simulink model "O4"  (R2020b)
settings: Solver=ode4  StartTime=0.0  StopTime=180  FixedStep=0.005  MinStep=0.001  RelTol=1e-3
model workspace (MAT data in the model file):
  Optimisation01_sdosession = sldodialogs.data.SessionData
  Optimisation01_sdosession.Version = '3.0'
  Optimisation01_sdosession.Data.ModelName = 'Optimisation01'
  Optimisation01_sdosession.Data.ToolType = 'ResponseOptimization'
  Optimisation01_sdosession.Data.GUIOptions.NoPromptClose = 0
  Optimisation01_sdosession.Data.Workspace.LocalWorkspace.DesignVars(1) = param.Continuous
  Optimisation01_sdosession.Data.Workspace.LocalWorkspace.DesignVars(1).Scale_ = 128
  Optimisation01_sdosession.Data.Workspace.LocalWorkspace.DesignVars(1).Size_ = [1 1]
  Optimisation01_sdosession.Data.Workspace.LocalWorkspace.DesignVars(1).Value_ = 50.1084192258
  Optimisation01_sdosession.Data.Workspace.LocalWorkspace.DesignVars(1).pID = paramid.Variable
  Optimisation01_sdosession.Data.Workspace.LocalWorkspace.DesignVars(1).pID.Name = 'Kd'
  Optimisation01_sdosession.Data.Workspace.LocalWorkspace.DesignVars(2) = param.Continuous
  Optimisation01_sdosession.Data.Workspace.LocalWorkspace.DesignVars(2).Scale_ = 8
  Optimisation01_sdosession.Data.Workspace.LocalWorkspace.DesignVars(2).Size_ = [1 1]
  Optimisation01_sdosession.Data.Workspace.LocalWorkspace.DesignVars(2).Value_ = 6.29568850936
  Optimisation01_sdosession.Data.Workspace.LocalWorkspace.DesignVars(2).pID = paramid.Variable
  Optimisation01_sdosession.Data.Workspace.LocalWorkspace.DesignVars(2).pID.Name = 'Ki'
  Optimisation01_sdosession.Data.Workspace.LocalWorkspace.DesignVars(3) = param.Continuous
  Optimisation01_sdosession.Data.Workspace.LocalWorkspace.DesignVars(3).Scale_ = 512
  Optimisation01_sdosession.Data.Workspace.LocalWorkspace.DesignVars(3).Size_ = [1 1]
  Optimisation01_sdosession.Data.Workspace.LocalWorkspace.DesignVars(3).Value_ = 364.260452278
  Optimisation01_sdosession.Data.Workspace.LocalWorkspace.DesignVars(3).pID = paramid.Variable
  Optimisation01_sdosession.Data.Workspace.LocalWorkspace.DesignVars(3).pID.Name = 'Kp'
  Optimisation01_sdosession.Data.Workspace.LocalWorkspace.ReqValues.Name = 'SignalProperty'
  Optimisation01_sdosession.Data.Workspace.LocalWorkspace.ReqValues.Type = 'min'
  Optimisation01_sdosession.Data.Workspace.LocalWorkspace.ReqValues.Value = 0.138601422932
  Optimisation01_sdosession.Data.Workspace.LocalWorkspace.ReqValues.DisplayValue = 0.138601422932
  Optimisation01_sdosession.Data.Workspace.LocalWorkspace.ReqValues_1.Name = 'SignalProperty'
  Optimisation01_sdosession.Data.Workspace.LocalWorkspace.ReqValues_1.Type = 'min'
  Optimisation01_sdosession.Data.Workspace.LocalWorkspace.ReqValues_1.Value = 0.264162161638
  Optimisation01_sdosession.Data.Workspace.LocalWorkspace.ReqValues_1.DisplayValue = 0.264162161638
  Optimisation01_sdosession.Data.Workspace.LocalWorkspace.Sig = Simulink.SimulationData.Signal
  Optimisation01_sdosession.Data.Workspace.LocalWorkspace.Sig.PortType = 'outport'
  Optimisation01_sdosession.Data.Workspace.LocalWorkspace.Sig.Version = 1
  Optimisation01_sdosession.Data.Workspace.LocalWorkspace.Sig.BlockPath = Simulink.SimulationData.BlockPath
  Optimisation01_sdosession.Data.Workspace.LocalWorkspace.Sig.BlockPath.path = {'Optimisation01/Sqrt'}
  Optimisation01_sdosession.Data.Workspace.LocalWorkspace.SignalProperty = sdo.requirements.SignalProperty
  Optimisation01_sdosession.Data.Workspace.LocalWorkspace.SignalProperty.sdo.requirements.Requirement.Data_ : srorequirement.functiondata (value not decoded)
  Optimisation01_sdosession.Data.Workspace.LocalWorkspace.SignalProperty.sdo.requirements.Requirement.Check_ = sdo.requirements.ScalarCheck
  Optimisation01_sdosession.Data.Workspace.HiddenWorkspace = []
  Optimisation01_sdosession.Data.ToolData.PlotManager.Plots(1).Class = 'sldoplots.TimePlot'
  Optimisation01_sdosession.Data.ToolData.PlotManager.Plots(1).Sources = {'Sig'}
  Optimisation01_sdosession.Data.ToolData.PlotManager.Plots(2).Class = 'sldoplots.IterPlot'
  Optimisation01_sdosession.Data.ToolData.PlotManager.Plots(2).Sources = {'SignalProperty'}
  Optimisation01_sdosession.Data.ToolData.PlotManager.Tiling : java.lang.String (value not decoded)
  Optimisation01_sdosession.Data.ToolData.DialogManager = []
  Optimisation01_sdosession.Data.ToolData.ResponseOptimization.Options = sdo.OptimizeOptions
  Optimisation01_sdosession.Data.ToolData.ResponseOptimization.Options.OptimizedModel = 'Optimisation01'
  Optimisation01_sdosession.Data.ToolData.ResponseOptimization.Options.Version = 2
  Optimisation01_sdosession.Data.ToolData.ResponseOptimization.GUIOptions.ModelTimeOut = Inf
  Optimisation01_sdosession.Data.ToolData.ResponseOptimization.GUIOptions.ComputeOperatingPoint = 0
  Optimisation01_sdosession.Data.ToolData.ResponseOptimization.GUIOptions.ShowProgress = 1
  Optimisation01_sdosession.Data.ToolData.ResponseOptimization.GUIOptions.ShowParamTrajectory = 1
  Optimisation01_sdosession.Data.ToolData.ResponseOptimization.GUIOptions.UpdatePlots = 1
  Optimisation01_sdosession.Data.ToolData.ResponseOptimization.GUIOptions.UpdateModel = 1
  Optimisation01_sdosession.Data.ToolData.ResponseOptimization.GUIOptions.UpdateDesign = 'overwrite'
  Optimisation01_sdosession.Data.ToolData.ResponseOptimization.GUIOptions.SaveReport = 0
  Optimisation01_sdosession.Data.ToolData.ResponseOptimization.GUIOptions.SaveRequirementValue = 1
  Optimisation01_sdosession.Data.ToolData.ResponseOptimization.LinOptions = linearize.LinearizeOptions
  Optimisation01_sdosession.Data.ToolData.ResponseOptimization.RequirementOperatingPointSetup = []
  Optimisation01_sdosession.Data.ToolData.ResponseOptimization.LocalRequirements.Requirement = 'SignalProperty'
  Optimisation01_sdosession.Data.ToolData.ResponseOptimization.LocalRequirements.Source = {'Sig'}
  Optimisation01_sdosession.Data.ToolData.ResponseOptimization.LocalRequirements.Selected = 1
  Optimisation01_sdosession.Data.ToolData.ResponseOptimization.BlockRequirements = struct([])
  Optimisation01_sdosession.Data.ToolData.ResponseOptimization.LocalExperiments = struct([])
  Optimisation01_sdosession.Data.ToolData.ResponseOptimization.Cost.Type = 'SSE'
  Optimisation01_sdosession.Data.ToolData.ResponseOptimization.Cost.Robust = 'off'
  Optimisation01_sdosession.Data.ToolData.ResponseOptimization.DesignVariables = 'DesignVars'
  Optimisation01_sdosession.Data.ToolData.ResponseOptimization.UncertainVariables = ''
  Optimisation01_sdosession.Data.ToolData.ResponseOptimization.DataToPlot = 'Sig'
values from neighbouring files (symbols this model uses):
  Kb = 0.4723    [O4.mat]
  Kd = 8.254    [O4.mat]
  Ki = 29.39    [O4.mat]
  Kp = 30.469    [O4.mat]
  Power = [0 0.134792669981 8.9180951627 7.77881648635 9.00749423422 8.96525793889 8.86751268571 15.7018632633 17.9613465432 18.9048532467 25.8479530412 34.4413156644 ... (50 elements, 50x1)]    [O4.mat]
  Throttle = [0 1 2.66666666667 3.44444444444 6.55555555556 8.11111111111 8.88888888889 13.6666666667 14.4444444444 15.2222222222 18.3333333333 21.5555555556 ... (50 elements, 50x1)]    [O4.mat]
  Thrust = [0 0.00386703849483 0.447248955951 0.381725752671 0.429816366755 0.448130327307 0.434268732353 0.786362880096 0.850043356053 0.907127881895 1.24377109743 1.5194958901 ... (50 elements, 50x1)]    [O4.mat]
undefined symbols (not defined in the file or in its folder): pulse, sawtooth
libraries: simulink x11, pid_lib x1, dspspect3 x1
settings Model: Creator=IR13  LastModifiedBy=IR13
settings SolverCC: ZeroCrossAlgorithm=Adaptive
settings DataIOCC: ReturnWorkspaceOutputsName=SDOSimTest_Log  Refine=2
settings OptimizationCC: DefaultUnderspecifiedDataType=single
settings DebuggingCC: IgnoredZcDiagnostic=none

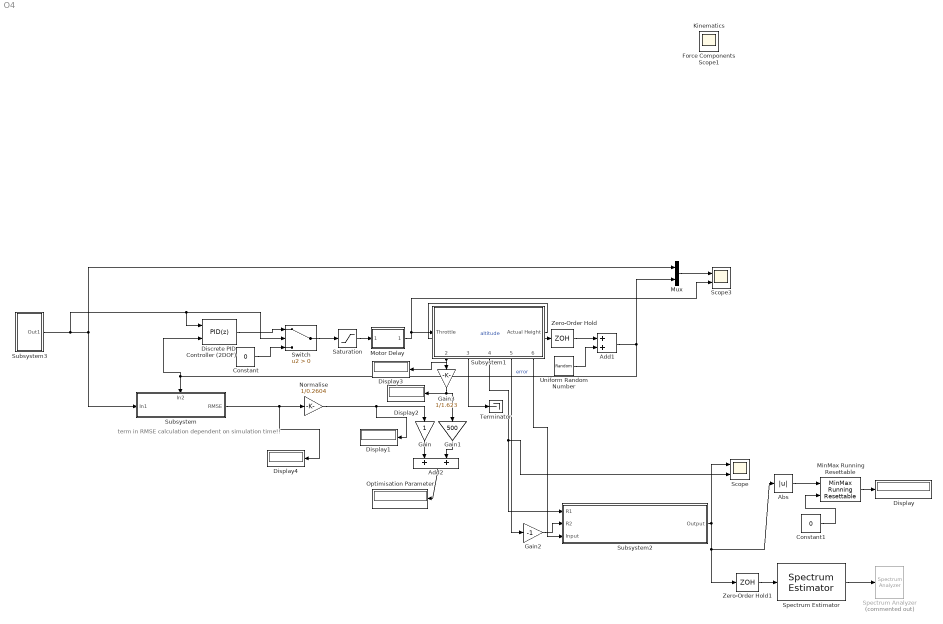
== system O4 ==
  note: term in RMSE calculation dependent on simulation time!!
  Abs : Abs
  Add1 : Sum
  Add2 : Sum
  Constant : Constant  Value=0
  Constant1 : Constant  Value=0
  Discrete PID Controller (2DOF) : pid_lib/PID Controller (2DOF)  Controller=PID  Form=Parallel  TimeDomain=Discrete-time  UseExternalTs=off  SampleTime=-1  IntegratorMethod=Forward Euler  FilterMethod=Forward Euler  ControllerParametersSource=internal  P=Kp  I=Ki  D=Kd  UseFilter=on  N=100  b=Kb  c=Kc  TunerSelectOption=Transfer Function Based (PID Tuner App)  InitialConditionSource=internal  InitialConditionForIntegrator=0  InitialConditionForFilter=0  DifferentiatorICPrevScaledInput=0  ExternalReset=none  TrackingMode=off  Kt=1  LimitOutput=off  SatLimitsSource=internal  UpperSaturationLimit=inf  LowerSaturationLimit=-inf  LinearizeAsGain=off  AntiWindupMode=none  Kb=1  POutMin=[]  POutMax=[]  IOutMin=[]  IOutMax=[]  DOutMin=[]  DOutMax=[]  NOutMin=[]  NOutMax=[]  bOutMin=[]  bOutMax=[]  cOutMin=[]  cOutMax=[]  SumOutMin=[]  SumOutMax=[]  SaturationOutMin=[]  SaturationOutMax=[]  PParamMin=[]  PParamMax=[]  IParamMin=[]  IParamMax=[]  DParamMin=[]  DParamMax=[]  NParamMin=[]  NParamMax=[]  bParamMin=[]  bParamMax=[]  cParamMin=[]  cParamMax=[]  KbParamMin=[]  KbParamMax=[]  KtParamMin=[]  KtParamMax=[]  KbOutMin=[]  KbOutMax=[]  KtOutMin=[]  KtOutMax=[]  IntegratorOutMin=[]  IntegratorOutMax=[]  FilterOutMin=[]  FilterOutMax=[]  SumI1OutMin=[]  SumI1OutMax=[]  SumI2OutMin=[]  SumI2OutMax=[]  SumI3OutMin=[]  SumI3OutMax=[]  SumI4OutMin=[]  SumI4OutMax=[]  SumDOutMin=[]  SumDOutMax=[]  Sum1OutMin=[]  Sum1OutMax=[]  Sum2OutMin=[]  Sum2OutMax=[]  Sum3OutMin=[]  Sum3OutMax=[]  DifferentiatorOutMin=[]  DifferentiatorOutMax=[]  FilterDiffOutCoefMin=[]  FilterDiffOutCoefMax=[]  ReciprocalOutMin=[]  ReciprocalOutMax=[]  SumDenOutMin=[]  SumDenOutMax=[]  SumNumOutMin=[]  SumNumOutMax=[]  DivideOutMin=[]  DivideOutMax=[]  UdiffTsProdOutMin=[]  UdiffTsProdOutMax=[]  NTsProdOutMin=[]  NTsProdOutMax=[]  UintegralTsProdOutMin=[]  UintegralTsProdOutMax=[]  UngainTsProdOutMin=[]  UngainTsProdOutMax=[]  IntegratorContinuousStateAttributes=''  IntegratorStateMustResolveToSignalObject=off  IntegratorRTWStateStorageClass=Auto  FilterContinuousStateAttributes=''  FilterStateMustResolveToSignalObject=off  FilterRTWStateStorageClass=Auto  ParallelPVariant=InternalParameters  IdealPVariant=Disabled  IVariant=InternalParameters  DVariant=InternalParameters  bVariant=InternalParameters  cVariant=InternalParameters  IntegratorVariant=Discrete  SatVariant=Disabled  AWVariant=Passthrough  PCopyVariant=Disabled  TRVariant=Disabled  FdbkBlocksVariant=Forward  IdealPFdbkVariant=Disabled  SatFdbkVariant=Disabled  DerivativeFilterVariant=ForwardEulerFilter  NVariant=InternalParameters  NCopyVariant=Disabled  FilterICVariant=InternalICsFilter  IntegratorICVariant=InternalICs  ExternalResetVariant=Disabled  TRSumVariant=Passthrough  SumFdbkVariant=Disabled  SumVariant=Sum_PID  TsampFilterVariant=InternalTs  TsampNgainVariant=Passthrough  TsampIntegralVariant=Passthrough  ExternalSaturationOutDataTypeStr=Inherit: Same as second input
      settings: SourceProductBaseCode=SL
  Display{,1..4} (5 alike) : Display
      Display3 settings: Decimation=2
  Gain : Gain
  Gain1 : Gain  Gain=500
  Gain2 : Gain  Gain=-1
  Gain3 : Gain  Gain=1/1.623
  MinMax Running Resettable : simulink/Math Operations/MinMax Running Resettable  Function=max  vinit=0.0
  Motor Delay : Subsystem
  Mux : Mux  Inputs=2
  Normalise : Gain  Gain=1/0.2604
  Optimisation Parameter : Display
  Saturation : Saturate  UpperLimit=100  LowerLimit=0
  Scope : Scope  NumInputPorts=2
  Scope3 : Scope  NumInputPorts=2
  Spectrum Analyzer : SpectrumAnalyzer  Commented=on  IsFrequencyInputMode=1
  Spectrum Estimator : dspspect3/Spectrum Estimator  Method=Filter bank  NumTapsPerBand=12  SpectrumType=Power  FrequencyResolutionMethod=Auto  FilterBankResolutionMethod=Auto  RBW=5  WindowLength=1024  FrequencyBandsSource=Same as input frame size  FrequencyBands=1024  FFTLengthSource=Auto  FFTLength=1024  InheritSampleRate=on  SampleRate=44100  Window=Hann  SidelobeAttenuation=60  AveragingMethod=Running  SpectralAverages=1  ForgettingFactorPort=off  ForgettingFactor=0.9  Overlap=0  ReferenceLoad=1  FrequencyRange=Centered  PowerUnits=dBm  OutputMaxHoldSpectrum=off  OutputMinHoldSpectrum=off  OutputFrequencyVector=off  OutputRBW=off  SimulateUsing=Code generation
      settings: SourceProductBaseCode=DS
  Subsystem : Subsystem
      settings: PortSchema="{\"entries\":[{\"content\":{\"sides\":[{\"content\":{\"connectorIds\":[\"In1\"]},\"type\":\"ConnectorPlacement.EquallySpacedRectSide\",\"uuid\":\"b7ba5938-330c-4f28-92b4-2f3c918ff7d8\"},{\"content\":{\"connectorIds\":[\"Out1\"],\"side\":\"RIGHT\"},\"type\":\"ConnectorPlacement.EquallySpacedRectSide\",\"uuid\":\"916077a3-2ae0-4004-b2f6-79a41e268964\"},{\"content\":{\"connectorIds\":[\"In2\"],\"side\":\"TOP\"},\"type\":\"ConnectorPlacement.EquallySpacedRectSide\",\"uuid\":\"773ac63e-b71f-4f33-b29a-efc56b3b32a1\"},{\"content\":{\"connectorIds\":[],\"side\":\"HIDDEN\"},\"type\":\"ConnectorPlacement.EquallySpacedRectSide\",\"uuid\":\"40b03bbd-b4d9-4aed-8815-b3f0a6a4b3fe\"}]},\"type\":\"ConnectorPlacement.EquallySpacedConnector\",\"uuid\":\"e2dbb7ef-3b06-4730-a49f-aaf53da408af\"}],\"packageUris\":[\"http://schema.mathworks.com/mf0/Connector/R2020b\"],\"version\":\"1.0\"}"
  Subsystem1 : Subsystem
      settings: PortSchema="{\"entries\":[{\"content\":{\"sides\":[{\"content\":{\"connectorIds\":[\"In1\"]},\"type\":\"ConnectorPlacement.EquallySpacedRectSide\",\"uuid\":\"75f601ae-023f-4048-a4e0-7d9af0b49ee8\"},{\"content\":{\"connectorIds\":[\"Out1\"],\"side\":\"RIGHT\"},\"type\":\"ConnectorPlacement.EquallySpacedRectSide\",\"uuid\":\"0fca52f4-072d-4867-9452-1b2aad1918f5\"},{\"content\":{\"connectorIds\":[],\"side\":\"TOP\"},\"type\":\"ConnectorPlacement.EquallySpacedRectSide\",\"uuid\":\"c12a021f-cc73-4ce4-a610-33f261e30a32\"},{\"content\":{\"connectorIds\":[\"Out2\",\"Out3\",\"Out4\",\"Out5\",\"Out6\"],\"side\":\"BOTTOM\"},\"type\":\"ConnectorPlacement.EquallySpacedRectSide\",\"uuid\":\"2a436ad0-e024-44cf-b443-7498d887a6e8\"},{\"content\":{\"connectorIds\":[],\"side\":\"HIDDEN\"},\"type\":\"ConnectorPlacement.EquallySpacedRectSide\",\"uuid\":\"c5caffb6-45a6-45f2-9e6d-3216775b27f4\"}]},\"type\":\"ConnectorPlacement.EquallySpacedConnector\",\"uuid\":\"4f32a242-49b5-4c90-b6e6-273e4e091971\"}],\"packageUris\":[\"http://schema.mathworks.com/mf0/Connector/R2020b\"],\"version\":\"1.0\"}"
  Subsystem2 : Subsystem
  Subsystem3 : Subsystem
  Switch : Switch  Criteria=u2 > Threshold
  Terminator : Terminator
  Uniform Random Number : UniformRandomNumber  Minimum=-0.01  Maximum=+0.01  SampleTime=0.005
  Zero-Order Hold : ZeroOrderHold  SampleTime=0.005
  Zero-Order Hold1 : ZeroOrderHold  SampleTime=0.005
  Force Components : Scope
  Kinematics : Scope
  Scope1 : Scope
  wires:
  Saturation/1 -> Motor Delay/1(Input)
  Add1/1 -> Subsystem/2(In2), Discrete PID Controller (2DOF)/2, Mux/2  "error"
  Subsystem3/1(Out1) -> Discrete PID Controller (2DOF)/1, Switch/2, Subsystem/1(In1), Mux/1
  Subsystem1/1(Actual Height) -> Zero-Order Hold/1  "altitude"
  Switch/1 -> Saturation/1
  Mux/1 -> Scope3/1
  Subsystem1/2(Total Energy) -> Display3/1, Gain3/1
  Add2/1 -> Optimisation Parameter/1
  Zero-Order Hold/1 -> Add1/1
  Uniform Random Number/1 -> Add1/2
  Subsystem/1(RMSE) -> Display4/1, Normalise/1
  Gain/1 -> Add2/1
  Gain1/1 -> Add2/2
  Discrete PID Controller (2DOF)/1 -> Switch/1
  Constant/1 -> Switch/3
  Subsystem1/5(Mounting Point Dynamic Load) -> Gain2/1
  Subsystem1/4(Thrust Point Dynamic Load) -> Subsystem2/1(R1), Scope/2
  Motor Delay/1(Output) -> Scope3/2, Subsystem1/1(Throttle)
  Subsystem1/3(Static Load P) -> Terminator/1
  Gain2/1 -> Subsystem2/2(R2)
  Subsystem2/1(Output) -> Zero-Order Hold1/1, Abs/1, Scope/1
  Zero-Order Hold1/1 -> Spectrum Estimator/1
  Spectrum Estimator/1 -> Spectrum Analyzer/1
  MinMax Running Resettable/1 -> Display/1
  Constant1/1 -> MinMax Running Resettable/2
  Normalise/1 -> Display1/1, Gain/1
  Abs/1 -> MinMax Running Resettable/1
  Subsystem1/6(Inertial Mass) -> Subsystem2/3(Input)
  Gain3/1 -> Gain1/1, Display2/1

== system O4/Motor Delay ==
  Input : Inport
  Rate Limiter : RateLimiter  RisingSlewLimit=166.7  FallingSlewLimit=-166.7  SampleTimeMode=inherited
  Scope3 : Scope  NumInputPorts=2
  Output : Outport
  wires:
  Input/1 -> Scope3/1, Rate Limiter/1
  Rate Limiter/1 -> Scope3/2, Output/1

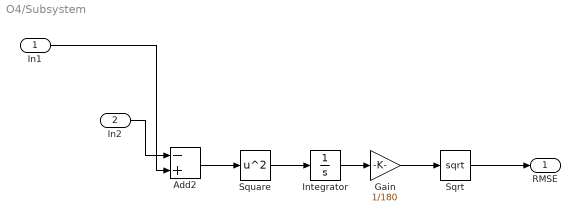
== system O4/Subsystem ==
  In1 : Inport
  In2 : Inport  Port=2
  Add2 : Sum  Inputs=-+
  Gain : Gain  Gain=1/180
  Integrator : Integrator
  Sqrt : Sqrt  SaturateOnIntegerOverflow=on
  Square : Math  Operator=square  SaturateOnIntegerOverflow=on
  RMSE : Outport
  wires:
  In2/1 -> Add2/1
  In1/1 -> Add2/2
  Add2/1 -> Square/1
  Gain/1 -> Sqrt/1
  Sqrt/1 -> RMSE/1
  Integrator/1 -> Gain/1
  Square/1 -> Integrator/1

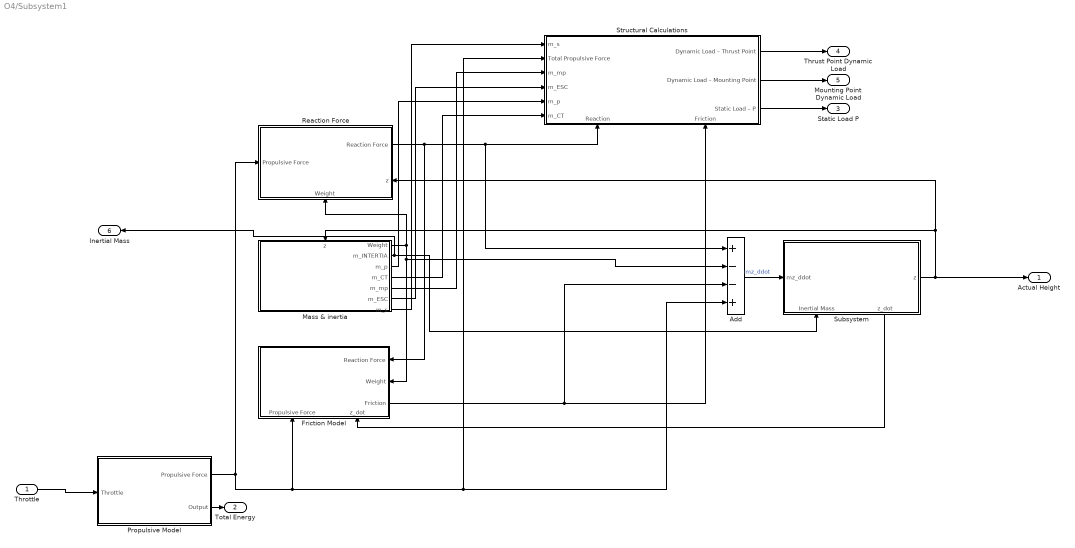
== system O4/Subsystem1 ==
  Throttle : Inport
  Add : Sum  Inputs=+--+
  Friction Model : Subsystem
      settings: PortSchema="{\"entries\":[{\"content\":{\"sides\":[{\"content\":{\"connectorIds\":[]},\"type\":\"ConnectorPlacement.EquallySpacedRectSide\",\"uuid\":\"1b3e095a-62ff-489c-96d9-63a8a1a842c7\"},{\"content\":{\"connectorIds\":[\"In3\",\"In4\",\"Out1\"],\"side\":\"RIGHT\"},\"type\":\"ConnectorPlacement.EquallySpacedRectSide\",\"uuid\":\"2aa3988f-f37b-48ca-a763-ece382c29199\"},{\"content\":{\"connectorIds\":[],\"side\":\"TOP\"},\"type\":\"ConnectorPlacement.EquallySpacedRectSide\",\"uuid\":\"ef7ffbd1-84d2-4291-ae41-90f24840b975\"},{\"content\":{\"connectorIds\":[\"In1\",\"In2\"],\"side\":\"BOTTOM\"},\"type\":\"ConnectorPlacement.EquallySpacedRectSide\",\"uuid\":\"ca187e87-455c-44d4-b2d5-496c3fe29e76\"},{\"content\":{\"connectorIds\":[],\"side\":\"HIDDEN\"},\"type\":\"ConnectorPlacement.EquallySpacedRectSide\",\"uuid\":\"11859c76-ab54-4977-b256-12d02241e5aa\"}]},\"type\":\"ConnectorPlacement.EquallySpacedConnector\",\"uuid\":\"162037a6-f725-4d16-a5f0-9112b8e8c48a\"}],\"packageUris\":[\"http://schema.mathworks.com/mf0/Connector/R2020b\"],\"version\":\"1.0\"}"
  Mass & inertia : Subsystem
      settings: PortSchema="{\"entries\":[{\"content\":{\"sides\":[{\"content\":{\"connectorIds\":[]},\"type\":\"ConnectorPlacement.EquallySpacedRectSide\",\"uuid\":\"1399d11e-8fed-4a75-a6ac-2b525e4dbe81\"},{\"content\":{\"connectorIds\":[\"Out1\",\"Out2\",\"Out3\",\"Out4\",\"Out5\",\"Out6\",\"Out7\"],\"side\":\"RIGHT\"},\"type\":\"ConnectorPlacement.EquallySpacedRectSide\",\"uuid\":\"2e2e7a23-dcb2-4001-96a5-c1562d5723c6\"},{\"content\":{\"connectorIds\":[\"In1\"],\"side\":\"TOP\"},\"type\":\"ConnectorPlacement.EquallySpacedRectSide\",\"uuid\":\"b0373260-5e1a-43dd-bca8-24421c20e285\"},{\"content\":{\"connectorIds\":[],\"side\":\"HIDDEN\"},\"type\":\"ConnectorPlacement.EquallySpacedRectSide\",\"uuid\":\"35e9db29-fffd-4860-9f0e-8f51711f4d01\"}]},\"type\":\"ConnectorPlacement.EquallySpacedConnector\",\"uuid\":\"39bd9006-0e99-41e8-8a89-05408a55c646\"}],\"packageUris\":[\"http://schema.mathworks.com/mf0/Connector/R2020b\"],\"version\":\"1.0\"}"
  Propulsive Model : Subsystem
  Reaction Force : Subsystem
      settings: PortSchema="{\"entries\":[{\"content\":{\"sides\":[{\"content\":{\"connectorIds\":[\"In1\"]},\"type\":\"ConnectorPlacement.EquallySpacedRectSide\",\"uuid\":\"1e35d603-08eb-402b-a2de-16d799202cf1\"},{\"content\":{\"connectorIds\":[\"Out1\",\"In3\"],\"side\":\"RIGHT\"},\"type\":\"ConnectorPlacement.EquallySpacedRectSide\",\"uuid\":\"6309f8f8-5c50-477a-b178-9a414ecebc78\"},{\"content\":{\"connectorIds\":[],\"side\":\"TOP\"},\"type\":\"ConnectorPlacement.EquallySpacedRectSide\",\"uuid\":\"1075b443-bbcc-4bf5-9b05-7b44ecc9bacc\"},{\"content\":{\"connectorIds\":[\"In2\"],\"side\":\"BOTTOM\"},\"type\":\"ConnectorPlacement.EquallySpacedRectSide\",\"uuid\":\"9465d0d7-9803-4a37-84cd-7fa866de481e\"},{\"content\":{\"connectorIds\":[],\"side\":\"HIDDEN\"},\"type\":\"ConnectorPlacement.EquallySpacedRectSide\",\"uuid\":\"80b90c9b-51c1-4183-87d9-243ed5e6c391\"}]},\"type\":\"ConnectorPlacement.EquallySpacedConnector\",\"uuid\":\"514452d4-5b8b-4aa9-8f6a-f7d3b564ce33\"}],\"packageUris\":[\"http://schema.mathworks.com/mf0/Connector/R2020b\"],\"version\":\"1.0\"}"
  Structural Calculations : Subsystem
      settings: PortSchema="{\"entries\":[{\"content\":{\"sides\":[{\"content\":{\"connectorIds\":[\"In1\",\"In2\"]},\"type\":\"ConnectorPlacement.EquallySpacedRectSide\",\"uuid\":\"199d6d66-4bc4-41e3-b0cf-b6dc827b3d17\"},{\"content\":{\"connectorIds\":[],\"side\":\"RIGHT\"},\"type\":\"ConnectorPlacement.EquallySpacedRectSide\",\"uuid\":\"5b09a715-a2be-4d36-86f7-2f96b16fd4b0\"},{\"content\":{\"connectorIds\":[\"In3\",\"In4\",\"In5\",\"In6\",\"In7\",\"In8\"],\"side\":\"TOP\"},\"type\":\"ConnectorPlacement.EquallySpacedRectSide\",\"uuid\":\"3ddf6b27-deb7-497d-8ce5-284ef95acabf\"},{\"content\":{\"connectorIds\":[\"Out1\",\"Out2\",\"Out3\"],\"side\":\"BOTTOM\"},\"type\":\"ConnectorPlacement.EquallySpacedRectSide\",\"uuid\":\"f9ac2c84-6bf1-49b2-9fa2-045548cdafcb\"},{\"content\":{\"connectorIds\":[],\"side\":\"HIDDEN\"},\"type\":\"ConnectorPlacement.EquallySpacedRectSide\",\"uuid\":\"b2b3b527-e15f-4e0a-bc29-4016fdde6e55\"}]},\"type\":\"ConnectorPlacement.EquallySpacedConnector\",\"uuid\":\"a23a5bbd-6c9c-4107-9a3f-f8a3315f0cc8\"}],\"packageUris\":[\"http://schema.mathworks.com/mf0/Connector/R2020b\"],\"version\":\"1.0\"}"
  Subsystem : Subsystem
      settings: PortSchema="{\"entries\":[{\"content\":{\"sides\":[{\"content\":{\"connectorIds\":[\"In1\"]},\"type\":\"ConnectorPlacement.EquallySpacedRectSide\",\"uuid\":\"4280b032-842d-4d16-b8c5-b63b72592cbb\"},{\"content\":{\"connectorIds\":[\"Out1\"],\"side\":\"RIGHT\"},\"type\":\"ConnectorPlacement.EquallySpacedRectSide\",\"uuid\":\"e4e0b7b9-12b8-4ae8-8e3c-cb8798002b22\"},{\"content\":{\"connectorIds\":[],\"side\":\"TOP\"},\"type\":\"ConnectorPlacement.EquallySpacedRectSide\",\"uuid\":\"d9ed1db6-3da5-4dd5-916f-0a0888e518e7\"},{\"content\":{\"connectorIds\":[\"In2\",\"Out2\"],\"side\":\"BOTTOM\"},\"type\":\"ConnectorPlacement.EquallySpacedRectSide\",\"uuid\":\"d18e58c7-4d86-4b90-a916-d0a361083c2d\"},{\"content\":{\"connectorIds\":[],\"side\":\"HIDDEN\"},\"type\":\"ConnectorPlacement.EquallySpacedRectSide\",\"uuid\":\"56aebb37-ad12-4a95-93b1-0a5b21e6f2e4\"}]},\"type\":\"ConnectorPlacement.EquallySpacedConnector\",\"uuid\":\"f0e8b7a0-91bd-4506-81db-435517f4e301\"}],\"packageUris\":[\"http://schema.mathworks.com/mf0/Connector/R2020b\"],\"version\":\"1.0\"}"
  Actual Height : Outport
  Total Energy : Outport  Port=2
  Static Load P : Outport  Port=3
  Thrust Point Dynamic Load : Outport  Port=4
  Mounting Point Dynamic Load : Outport  Port=5
  Inertial Mass : Outport  Port=6
  wires:
  Reaction Force/1(Reaction Force) -> Add/1, Structural Calculations/1(Reaction), Friction Model/3(Reaction Force)
  Mass & inertia/2(m_INTERTIA) -> Inertial Mass/1, Subsystem/2(Inertial Mass)
  Throttle/1 -> Propulsive Model/1(Throttle)
  Subsystem/1(z) -> Actual Height/1, Reaction Force/3(z), Mass & inertia/1(z)
  Subsystem/2(z_dot) -> Friction Model/2(z_dot)
  Propulsive Model/1(Propulsive Force) -> Add/4, Structural Calculations/7(Total Propulsive Force), Friction Model/1(Propulsive Force), Reaction Force/1(Propulsive Force)
  Add/1 -> Subsystem/1(mz_ddot)  "mz_ddot"
  Mass & inertia/1(Weight) -> Friction Model/4(Weight), Add/2, Reaction Force/2(Weight)
  Friction Model/1(Friction) -> Add/3, Structural Calculations/2(Friction)
  Propulsive Model/2(Output) -> Total Energy/1
  Structural Calculations/1(Static Load – P) -> Static Load P/1
  Structural Calculations/3(Dynamic Load – Thrust Point) -> Thrust Point Dynamic Load/1
  Structural Calculations/2(Dynamic Load – Mounting Point) -> Mounting Point Dynamic Load/1
  Mass & inertia/3(m_p) -> Structural Calculations/4(m_p)
  Mass & inertia/4(m_CT) -> Structural Calculations/3("m_CT ")
  Mass & inertia/5(m_mp) -> Structural Calculations/6(m_mp)
  Mass & inertia/6(m_ESC) -> Structural Calculations/5(m_ESC)
  Mass & inertia/7(m_s) -> Structural Calculations/8(m_s)

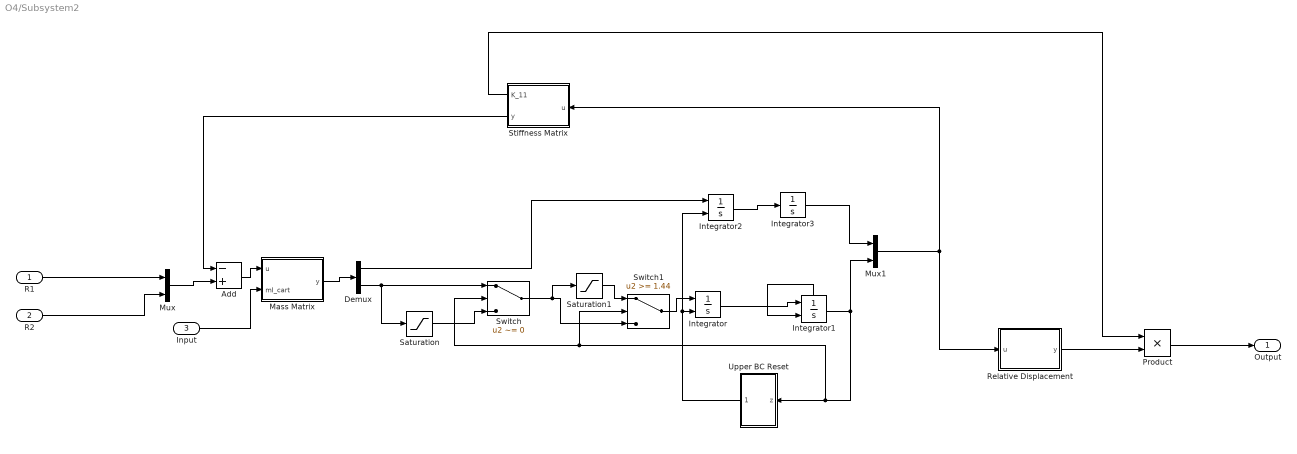
== system O4/Subsystem2 ==
  R1 : Inport
  R2 : Inport  Port=2
  Input : Inport  Port=3
  Add : Sum  Inputs=-+
  Demux : Demux  Outputs=2
  Integrator : Integrator  ExternalReset=falling
  Integrator1 : Integrator  ExternalReset=falling  ShowStatePort=on
  Integrator2 : Integrator  ExternalReset=falling
  Integrator3 : Integrator
  Mass Matrix : MATLAB Function  TreatAsAtomicUnit=on
  Mux : Mux  Inputs=2
  Mux1 : Mux  Inputs=2
  Product : Product
  Relative Displacement : MATLAB Function  TreatAsAtomicUnit=on
  Saturation : Saturate  UpperLimit=+inf  LowerLimit=0
  Saturation1 : Saturate  UpperLimit=0  LowerLimit=-inf
  Stiffness Matrix : MATLAB Function  TreatAsAtomicUnit=on
  Switch : Switch  Criteria=u2 ~= 0
  Switch1 : Switch  Threshold=1.44
  Upper BC Reset : Subsystem
  Output : Outport
  wires:
  Product/1 -> Output/1
  Relative Displacement/1(y) -> Product/2
  R2/1 -> Mux/2
  Stiffness Matrix/1(K_11) -> Product/1
  Mux/1 -> Add/2
  Stiffness Matrix/2(y) -> Add/1
  R1/1 -> Mux/1
  Add/1 -> Mass Matrix/1(u)
  Mass Matrix/1(y) -> Demux/1
  Demux/1 -> Integrator2/1
  Demux/2 -> Switch/1, Saturation/1
  Integrator/1 -> Integrator1/1
  Integrator1/State -> Integrator1/2
  Integrator3/1 -> Mux1/1
  Mux1/1 -> Relative Displacement/1(u), Stiffness Matrix/1(u)
  Integrator1/1 -> Switch/2, Switch1/2, Upper BC Reset/1(z), Mux1/2
  Upper BC Reset/1(Out1) -> Integrator2/2, Integrator/2
  Integrator2/1 -> Integrator3/1
  Switch/1 -> Saturation1/1, Switch1/3
  Saturation/1 -> Switch/3
  Switch1/1 -> Integrator/1
  Saturation1/1 -> Switch1/1
  Input/1 -> Mass Matrix/2(mI_cart)

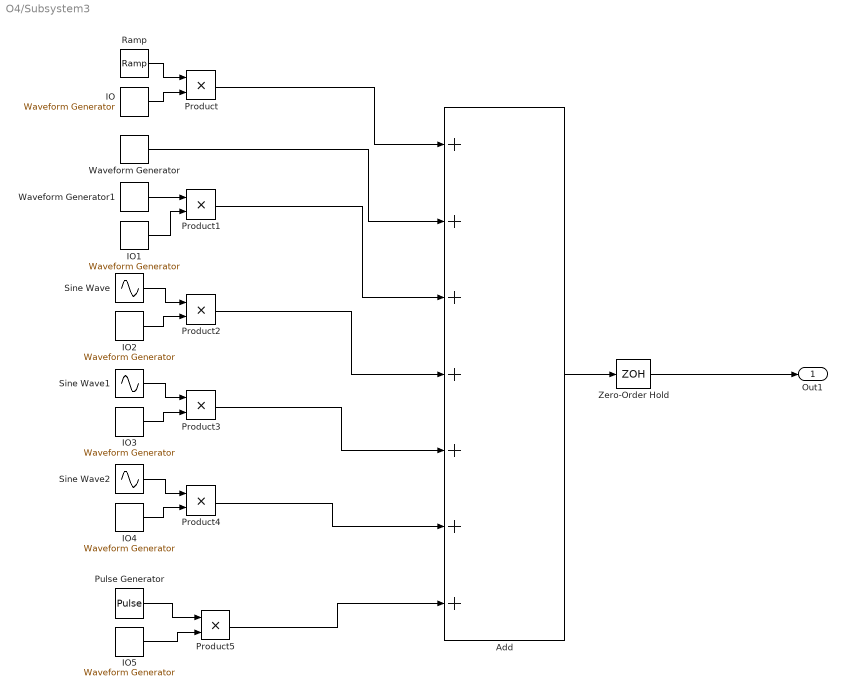
== system O4/Subsystem3 ==
  Add : Sum  Inputs=+++++++
  IO : simulink/Sources/Waveform Generator  OutMin=[]  OutMax=[]  OutDataTypeStr=double  SelectedSignal=1  Signals=pulse(1,0,5)  BlockNames=MultiportSwitch_13ecaae911a5496  SampleTime=0.1
  IO1 : simulink/Sources/Waveform Generator  OutMin=[]  OutMax=[]  OutDataTypeStr=double  SelectedSignal=1  Signals=pulse(1,68,20)  BlockNames=MultiportSwitch_8da1d444b60440f  SampleTime=0.1
  IO2 : simulink/Sources/Waveform Generator  OutMin=[]  OutMax=[]  OutDataTypeStr=double  SelectedSignal=1  Signals=pulse(1,92,20)  BlockNames=MultiportSwitch_a33517f4f9cd439  SampleTime=0.1
  IO3 : simulink/Sources/Waveform Generator  OutMin=[]  OutMax=[]  OutDataTypeStr=double  SelectedSignal=1  Signals=pulse(1,112.1,20)  BlockNames=MultiportSwitch_4da2be7ce746415  SampleTime=0.1
  IO4 : simulink/Sources/Waveform Generator  OutMin=[]  OutMax=[]  OutDataTypeStr=double  SelectedSignal=1  Signals=pulse(1,132.2,20)  BlockNames=MultiportSwitch_186056875532497  SampleTime=0.1
  IO5 : simulink/Sources/Waveform Generator  OutMin=[]  OutMax=[]  OutDataTypeStr=double  SelectedSignal=1  Signals=pulse(1,152.2,25)  BlockNames=MultiportSwitch_840003c23dc64bb  SampleTime=0.1
  Product{,1..5} (6 alike) : Product
  Pulse Generator : DiscretePulseGenerator  PulseType=Time based  Period=4  PulseWidth=40
  Ramp : simulink/Sources/Ramp  slope=0.2  start=0  InitialOutput=0
  Sine Wave : Sin  Amplitude=0.35  Bias=0.6  Frequency=2  Phase=0.6  SampleTime=0
  Sine Wave1 : Sin  Amplitude=0.5  Bias=0.6  Frequency=0.5  Phase=0.6  SampleTime=0
  Sine Wave2 : Sin  Amplitude=0.1  Bias=0.6  Frequency=0.3  Phase=0.6  SampleTime=0
  Waveform Generator : simulink/Sources/Waveform Generator  OutMin=[]  OutMax=[]  OutDataTypeStr=double  SelectedSignal=1  Signals=pulse(1.44,10,5) + pulse(0.5,22,5) + pulse(0.2,35,9.995) + pulse(0.5,45,9.996) + pulse(1.2,55,10)  BlockNames=MultiportSwitch_9705515f1dd0407  SampleTime=0.005
  Waveform Generator1 : simulink/Sources/Waveform Generator  OutMin=[]  OutMax=[]  OutDataTypeStr=double  SelectedSignal=1  Signals=sawtooth(0.6,1, 0) + 0.7  BlockNames=MultiportSwitch_0bc234dcf7e84f6  SampleTime=0.005
  Zero-Order Hold : ZeroOrderHold  SampleTime=-1
  Out1 : Outport
  wires:
  Product4/1 -> Add/6
  Waveform Generator/1 -> Add/2
  IO/1 -> Product/2
  IO1/1 -> Product1/2
  Ramp/1 -> Product/1
  IO3/1 -> Product3/2
  Sine Wave2/1 -> Product4/1
  IO2/1 -> Product2/2
  Waveform Generator1/1 -> Product1/1
  Product3/1 -> Add/5
  Zero-Order Hold/1 -> Out1/1
  IO5/1 -> Product5/2
  Sine Wave/1 -> Product2/1
  Add/1 -> Zero-Order Hold/1
  Product/1 -> Add/1
  Pulse Generator/1 -> Product5/1
  IO4/1 -> Product4/2
  Sine Wave1/1 -> Product3/1
  Product1/1 -> Add/3
  Product2/1 -> Add/4
  Product5/1 -> Add/7

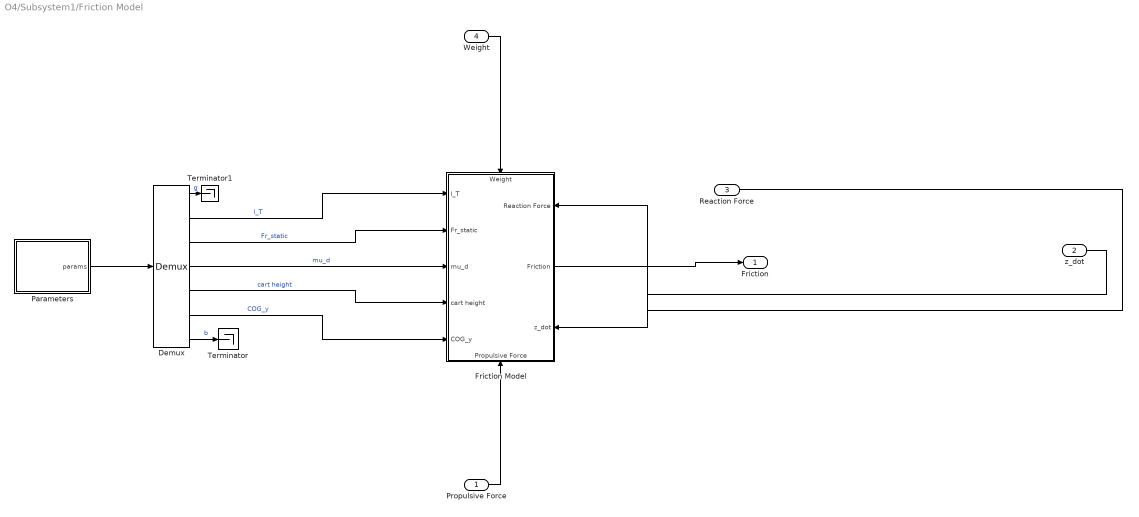
== system O4/Subsystem1/Friction Model ==
  Propulsive Force : Inport
  z_dot : Inport  Port=2
  Reaction Force : Inport  Port=3
  Weight : Inport  Port=4
  Demux : Demux  Outputs=7
  Friction Model : Subsystem
      settings: PortSchema="{\"entries\":[{\"content\":{\"sides\":[{\"content\":{\"connectorIds\":[\"In1\",\"In2\",\"In3\",\"In4\",\"In5\"]},\"type\":\"ConnectorPlacement.EquallySpacedRectSide\",\"uuid\":\"b80da770-fdb0-4d6f-bea5-94e06f2afa04\"},{\"content\":{\"connectorIds\":[\"In8\",\"Out1\",\"In9\"],\"side\":\"RIGHT\"},\"type\":\"ConnectorPlacement.EquallySpacedRectSide\",\"uuid\":\"44cc0c5b-7bc2-4d7d-ab9c-4e4237bff03f\"},{\"content\":{\"connectorIds\":[\"In6\"],\"side\":\"TOP\"},\"type\":\"ConnectorPlacement.EquallySpacedRectSide\",\"uuid\":\"d8cf9831-f5c9-4bfd-8650-bb94040859dc\"},{\"content\":{\"connectorIds\":[\"In7\"],\"side\":\"BOTTOM\"},\"type\":\"ConnectorPlacement.EquallySpacedRectSide\",\"uuid\":\"5dc8ad5a-b457-4b35-ae96-3ded03a76763\"},{\"content\":{\"connectorIds\":[],\"side\":\"HIDDEN\"},\"type\":\"ConnectorPlacement.EquallySpacedRectSide\",\"uuid\":\"8dab3da8-cd9e-407c-8850-bafd2d7a131e\"}]},\"type\":\"ConnectorPlacement.EquallySpacedConnector\",\"uuid\":\"d0f16782-5cb8-4cea-b1e1-f78879901c5f\"}],\"packageUris\":[\"http://schema.mathworks.com/mf0/Connector/R2020b\"],\"version\":\"1.0\"}"
  Parameters : MATLAB Function  TreatAsAtomicUnit=on
  Terminator : Terminator
  Terminator1 : Terminator
  Friction : Outport
  wires:
  Demux/7 -> Terminator/1  "b"
  Reaction Force/1 -> Friction Model/8(Reaction Force)
  Demux/1 -> Terminator1/1  "g"
  Propulsive Force/1 -> Friction Model/7(Propulsive Force)
  Demux/2 -> Friction Model/1(l_T)  "l_T"
  Friction Model/1(Friction) -> Friction/1
  Weight/1 -> Friction Model/6(Weight)
  Demux/3 -> Friction Model/2(Fr_static)  "Fr_static"
  Parameters/1(params) -> Demux/1
  Demux/4 -> Friction Model/3(mu_d)  "mu_d"
  z_dot/1 -> Friction Model/9(z_dot)
  Demux/5 -> Friction Model/4(cart height)  "cart height"
  Demux/6 -> Friction Model/5(COG_y)  "COG_y"

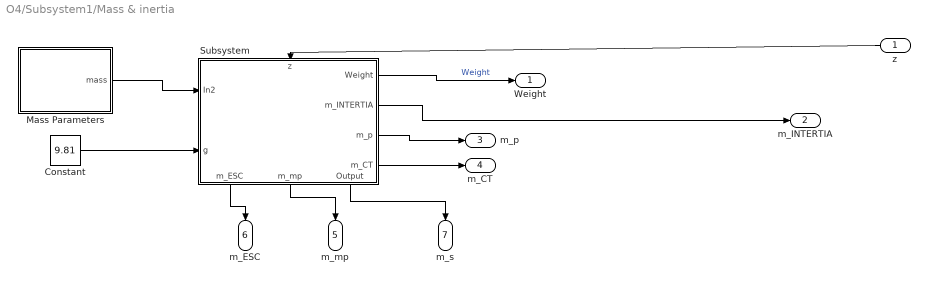
== system O4/Subsystem1/Mass & inertia ==
  z : Inport
  Constant : Constant  Value=9.81
  Mass Parameters : MATLAB Function  TreatAsAtomicUnit=on
  Subsystem : Subsystem
      settings: PortSchema="{\"entries\":[{\"content\":{\"sides\":[{\"content\":{\"connectorIds\":[\"In1\",\"In2\"]},\"type\":\"ConnectorPlacement.EquallySpacedRectSide\",\"uuid\":\"22ad1645-0c4a-4eab-a942-e35708909bc2\"},{\"content\":{\"connectorIds\":[\"Out1\",\"Out2\",\"Out3\",\"Out4\"],\"side\":\"RIGHT\"},\"type\":\"ConnectorPlacement.EquallySpacedRectSide\",\"uuid\":\"049dc02c-af21-4242-96fd-198a717a970b\"},{\"content\":{\"connectorIds\":[\"In3\"],\"side\":\"TOP\"},\"type\":\"ConnectorPlacement.EquallySpacedRectSide\",\"uuid\":\"a1727784-13c5-452f-b8c4-4da743b82409\"},{\"content\":{\"connectorIds\":[\"Out5\",\"Out6\",\"Out7\"],\"side\":\"BOTTOM\"},\"type\":\"ConnectorPlacement.EquallySpacedRectSide\",\"uuid\":\"0977ed5c-83b4-4037-9cbd-ef510b1b93e7\"},{\"content\":{\"connectorIds\":[],\"side\":\"HIDDEN\"},\"type\":\"ConnectorPlacement.EquallySpacedRectSide\",\"uuid\":\"a08d060c-4763-496d-ac54-202c99d24543\"}]},\"type\":\"ConnectorPlacement.EquallySpacedConnector\",\"uuid\":\"dcd15304-2046-43f2-990d-e6438030fbb8\"}],\"packageUris\":[\"http://schema.mathworks.com/mf0/Connector/R2020b\"],\"version\":\"1.0\"}"
  Weight : Outport
  m_INTERTIA : Outport  Port=2
  m_p : Outport  Port=3
  m_CT : Outport  Port=4
  m_mp : Outport  Port=5
  m_ESC : Outport  Port=6
  m_s : Outport  Port=7
  wires:
  Subsystem/2(m_INTERTIA) -> m_INTERTIA/1
  Constant/1 -> Subsystem/2(g)
  Subsystem/1(Weight) -> Weight/1  "Weight"
  z/1 -> Subsystem/3(z)
  Mass Parameters/1(mass) -> Subsystem/1(In2)
  Subsystem/3(m_p) -> m_p/1
  Subsystem/4(m_CT) -> m_CT/1
  Subsystem/5(m_ESC) -> m_ESC/1
  Subsystem/6(m_mp) -> m_mp/1
  Subsystem/7(Output) -> m_s/1

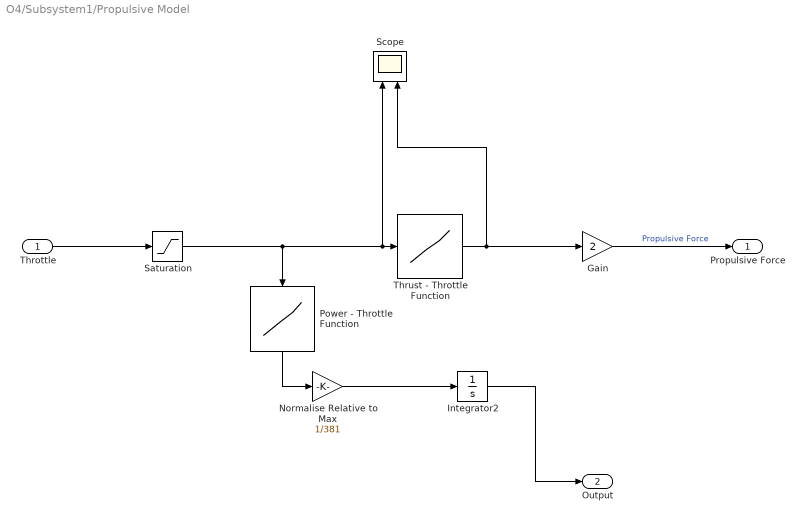
== system O4/Subsystem1/Propulsive Model ==
  Throttle : Inport
  Gain : Gain  Gain=2
  Integrator2 : Integrator
  Normalise Relative to Max : Gain  Gain=1/381
  Power - Throttle Function : Lookup_n-D  NumberOfTableDimensions=1  BreakpointsForDimension1=Throttle  BreakpointsForDimension2=[1:3]  Table=Power  ExtrapMethod=Clip  InternalRulePriority=Speed  RndMeth=Simplest  InputSameDT=on
  Saturation : Saturate  UpperLimit=100  LowerLimit=0
  Scope : Scope  NumInputPorts=2
  Thrust - Throttle Function : Lookup_n-D  NumberOfTableDimensions=1  BreakpointsForDimension1=Throttle  BreakpointsForDimension2=[1:3]  Table=Thrust  ExtrapMethod=Clip  DiagnosticForOutOfRangeInput=Warning  InternalRulePriority=Speed  RndMeth=Simplest  InputSameDT=on
  Propulsive Force : Outport
  Output : Outport  Port=2
  wires:
  Integrator2/1 -> Output/1
  Thrust - Throttle Function/1 -> Gain/1, Scope/2
  Power - Throttle Function/1 -> Normalise Relative to Max/1
  Gain/1 -> Propulsive Force/1  "Propulsive Force"
  Throttle/1 -> Saturation/1
  Saturation/1 -> Scope/1, Thrust - Throttle Function/1, Power - Throttle Function/1
  Normalise Relative to Max/1 -> Integrator2/1

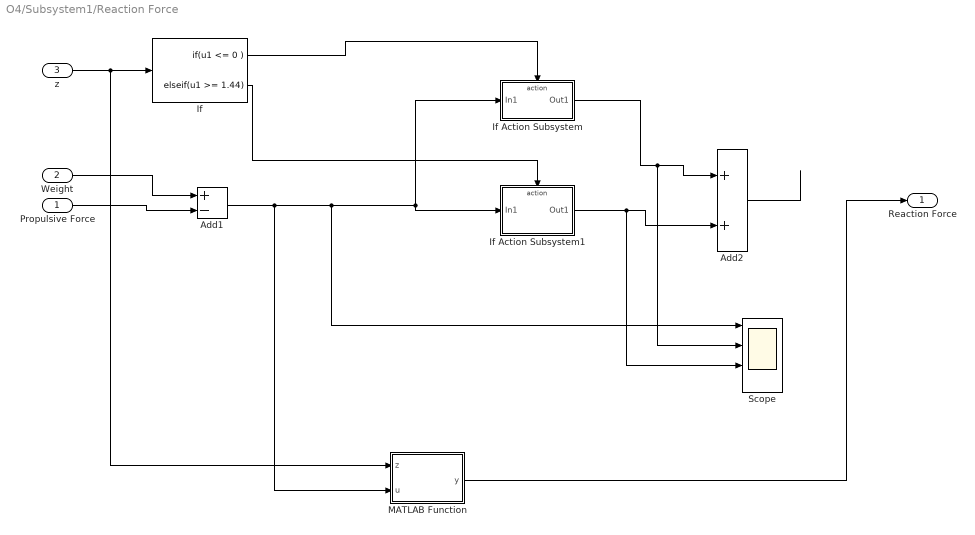
== system O4/Subsystem1/Reaction Force ==
  Propulsive Force : Inport
  Weight : Inport  Port=2
  z : Inport  Port=3
  Add1 : Sum  Inputs=+-
  Add2 : Sum
  If : If  IfExpression=u1 <= 0  ElseIfExpressions=u1 >= 1.44  ShowElse=off
  If Action Subsystem : Subsystem  TreatAsAtomicUnit=on
  If Action Subsystem1 : Subsystem  TreatAsAtomicUnit=on
  MATLAB Function : MATLAB Function  TreatAsAtomicUnit=on
  Scope : Scope  NumInputPorts=4
  Reaction Force : Outport
  wires:
  Weight/1 -> Add1/1
  If Action Subsystem1/1(Out1) -> Scope/3, Add2/2
  z/1 -> MATLAB Function/1(z), If/1
  Add2/1 -> ?
  If/2 -> If Action Subsystem1/Action
  Propulsive Force/1 -> Add1/2
  If Action Subsystem/1(Out1) -> Scope/2, Add2/1
  If/1 -> If Action Subsystem/Action
  Add1/1 -> MATLAB Function/2(u), Scope/1, If Action Subsystem1/1(In1), If Action Subsystem/1(In1)
  MATLAB Function/1(y) -> Reaction Force/1

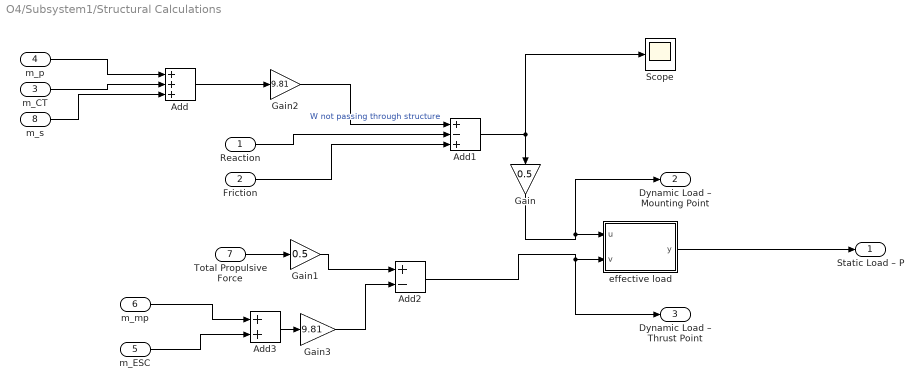
== system O4/Subsystem1/Structural Calculations ==
  Reaction : Inport
  Friction : Inport  Port=2
  "m_CT " : Inport  Port=3
  m_p : Inport  Port=4
  m_ESC : Inport  Port=5
  m_mp : Inport  Port=6
  Total Propulsive Force : Inport  Port=7
  m_s : Inport  Port=8
  Add : Sum  Inputs=+++
  Add1 : Sum  Inputs=+-+
  Add2 : Sum  Inputs=+-
  Add3 : Sum
  Gain : Gain  Gain=0.5
  Gain1 : Gain  Gain=0.5
  Gain2 : Gain  Gain=9.81
  Gain3 : Gain  Gain=9.81
  Scope : Scope
  "effective load " : MATLAB Function  TreatAsAtomicUnit=on
  Static Load – P : Outport
  Dynamic Load – Mounting Point : Outport  Port=2
  Dynamic Load – Thrust Point : Outport  Port=3
  wires:
  Total Propulsive Force/1 -> Gain1/1
  Friction/1 -> Add1/3
  Reaction/1 -> Add1/2
  Add1/1 -> Gain/1, Scope/1
  Add/1 -> Gain2/1
  m_mp/1 -> Add3/1
  Add2/1 -> "effective load "/2(v), Dynamic Load – Thrust Point/1
  m_ESC/1 -> Add3/2
  Add3/1 -> Gain3/1
  Gain/1 -> "effective load "/1(u), Dynamic Load – Mounting Point/1
  "effective load "/1(y) -> Static Load – P/1
  m_p/1 -> Add/1
  "m_CT "/1 -> Add/2
  Gain1/1 -> Add2/1
  Gain2/1 -> Add1/1  "W not passing through structure"
  Gain3/1 -> Add2/2
  m_s/1 -> Add/3

== system O4/Subsystem1/Subsystem ==
  mz_ddot : Inport
  Inertial Mass : Inport  Port=2
  Divide2 : Product  Inputs=/*
  Integrator : Integrator  ExternalReset=falling
  Integrator1 : Integrator  ExternalReset=falling  ShowStatePort=on
  Upper BC Reset : Subsystem
  z : Outport
  z_dot : Outport  Port=2
  wires:
  mz_ddot/1 -> Divide2/2
  Upper BC Reset/1(Out1) -> Integrator/2
  Inertial Mass/1 -> Divide2/1
  Divide2/1 -> Integrator/1  "z_ddot"
  Integrator1/State -> Integrator1/2
  Integrator1/1 -> Upper BC Reset/1(z), z/1  "z"
  Integrator/1 -> z_dot/1, Integrator1/1  "z_dot"

== system O4/Subsystem2/Upper BC Reset ==
  z : Inport
  Add1 : Sum  Inputs=+-
  Constant : Constant  Value=1.44
  Switch : Switch  Criteria=u2 > Threshold  Threshold=0.72
  Out1 : Outport
  wires:
  Add1/1 -> Switch/1
  Switch/1 -> Out1/1
  z/1 -> Add1/2, Switch/3, Switch/2
  Constant/1 -> Add1/1

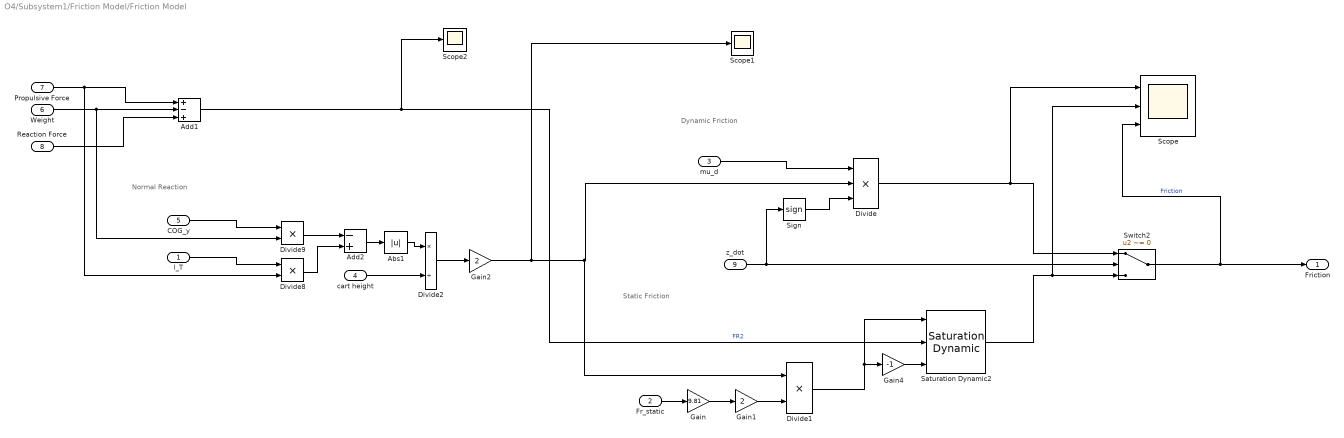
== system O4/Subsystem1/Friction Model/Friction Model ==
  note: Static Friction
  note: Dynamic Friction
  note: Normal Reaction
  l_T : Inport
  Fr_static : Inport  Port=2
  mu_d : Inport  Port=3
  cart height : Inport  Port=4
  COG_y : Inport  Port=5
  Weight : Inport  Port=6
  Propulsive Force : Inport  Port=7
  Reaction Force : Inport  Port=8
  z_dot : Inport  Port=9
  Abs1 : Abs
  Add1 : Sum  Inputs=+-+
  Add2 : Sum  Inputs=-+
  Divide : Product  Inputs=***
  Divide1 : Product  Inputs=**
  Divide2 : Product  Inputs=*/
  Divide8 : Product  Inputs=**
  Divide9 : Product  Inputs=**
  Gain : Gain  Gain=9.81
  Gain1 : Gain  Gain=2
  Gain2 : Gain  Gain=2
  Gain4 : Gain  Gain=-1
  Saturation Dynamic2 : simulink/Discontinuities/Saturation Dynamic  OutMin=[]  OutMax=[]  OutDataTypeStr=Inherit: Same as second input  OutDataType=fixdt(1, 16)  OutScaling=2^-10  DoSatur=off
  Scope : Scope  NumInputPorts=3
  Scope1 : Scope
  Scope2 : Scope
  Sign : Signum
  Switch2 : Switch  Criteria=u2 ~= 0
  Friction : Outport
  wires:
  Reaction Force/1 -> Add1/3
  Add2/1 -> Abs1/1
  COG_y/1 -> Divide9/1
  cart height/1 -> Divide2/2
  Divide2/1 -> Gain2/1
  Divide9/1 -> Add2/1
  Divide8/1 -> Add2/2
  Weight/1 -> Add1/2, Divide9/2
  Abs1/1 -> Divide2/1
  Propulsive Force/1 -> Divide8/2, Add1/1
  l_T/1 -> Divide8/1
  Switch2/1 -> Scope/3, Friction/1  "Friction"
  Divide/1 -> Scope/1, Switch2/1
  mu_d/1 -> Divide/1
  Sign/1 -> Divide/3
  z_dot/1 -> Sign/1, Switch2/2
  Add1/1 -> Scope2/1, Saturation Dynamic2/2  "FR2"
  Saturation Dynamic2/1 -> Scope/2, Switch2/3
  Divide1/1 -> Saturation Dynamic2/1, Gain4/1
  Gain4/1 -> Saturation Dynamic2/3
  Fr_static/1 -> Gain/1
  Gain/1 -> Gain1/1
  Gain2/1 -> Scope1/1, Divide1/1, Divide/2
  Gain1/1 -> Divide1/2

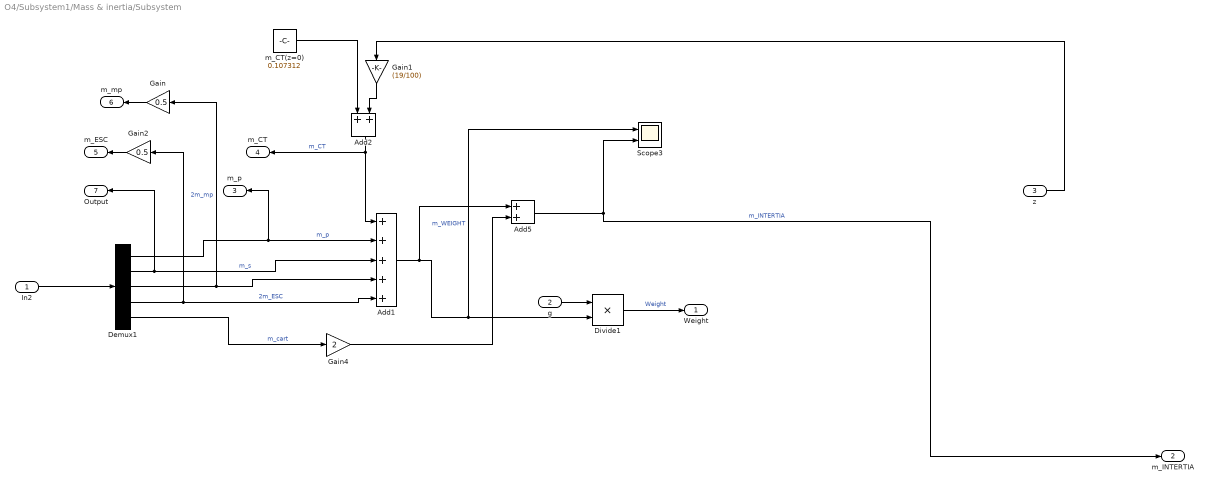
== system O4/Subsystem1/Mass & inertia/Subsystem ==
  In2 : Inport
  g : Inport  Port=2
  z : Inport  Port=3
  Add1 : Sum  Inputs=+++++
  Add2 : Sum
  Add5 : Sum
  Demux1 : Demux  Outputs=5
  Divide1 : Product  Inputs=**
  Gain : Gain  Gain=0.5
  Gain1 : Gain  Gain=(19/100)
  Gain2 : Gain  Gain=0.5
  Gain4 : Gain  Gain=2
  Scope3 : Scope  NumInputPorts=2
  m_CT(z=0) : Constant  Value=0.107312
  Weight : Outport
  m_INTERTIA : Outport  Port=2
  m_p : Outport  Port=3
  m_CT : Outport  Port=4
  m_ESC : Outport  Port=5
  m_mp : Outport  Port=6
  Output : Outport  Port=7
  wires:
  Demux1/5 -> Gain4/1  "m_cart"
  Demux1/2 -> Output/1, Add1/3  "m_s"
  Demux1/1 -> m_p/1, Add1/2  "m_p"
  Divide1/1 -> Weight/1  "Weight"
  Add2/1 -> Add1/1, m_CT/1  "m_CT"
  In2/1 -> Demux1/1
  Gain4/1 -> Add5/2
  g/1 -> Divide1/1
  Gain1/1 -> Add2/2
  Add5/1 -> m_INTERTIA/1, Scope3/2  "m_INTERTIA"
  z/1 -> Gain1/1
  m_CT(z=0)/1 -> Add2/1
  Demux1/3 -> Gain/1, Add1/4  "2m_mp"
  Demux1/4 -> Gain2/1, Add1/5  "2m_ESC"
  Add1/1 -> Add5/1, Scope3/1, Divide1/2  "m_WEIGHT"
  Gain/1 -> m_mp/1
  Gain2/1 -> m_ESC/1

== system O4/Subsystem1/Reaction Force/If Action Subsystem ==
  In1 : Inport
  Action Port : ActionPort  ActionPortLabel=if(u1 <= 0 )
  Saturation : Saturate  UpperLimit=+inf  LowerLimit=0  LinearizeAsGain=off
  Out1 : Outport
  wires:
  In1/1 -> Saturation/1
  Saturation/1 -> Out1/1

== system O4/Subsystem1/Reaction Force/If Action Subsystem1 ==
  In1 : Inport
  Action Port : ActionPort  ActionPortLabel=elseif(u1 >= 1.44)
  Saturation : Saturate  UpperLimit=0  LowerLimit=-inf  LinearizeAsGain=off
  Out1 : Outport
  wires:
  In1/1 -> Saturation/1
  Saturation/1 -> Out1/1

== system O4/Subsystem1/Subsystem/Upper BC Reset ==
  z : Inport
  Add1 : Sum  Inputs=+-
  Constant : Constant  Value=1.44
  Switch : Switch  Criteria=u2 > Threshold  Threshold=0.72
  Out1 : Outport
  wires:
  Add1/1 -> Switch/1
  Switch/1 -> Out1/1
  z/1 -> Add1/2, Switch/3, Switch/2
  Constant/1 -> Add1/1

== matlab function O4/Subsystem1/Friction Model/Parameters ==
  data: params output
function params = fcn()

%raw parameters
g = 9.81;
lT = 34.568; %y position of thrust point [mm]
F_r_static = 0.13; %static friction force [kgf]
mu_d = 0.14; %dynamic friction coefficient 
cart_height = 210.4; %[mm]
CoG_y = 20.0579; %%[mm]
b = 0.2; %damping constant

params = [g;lT;F_r_static; mu_d; cart_height;CoG_y;b];

== matlab function O4/Subsystem1/Structural Calculations/effective load  ==
  data: u input; y output; v input
function y = fcn(u,v)

if u * v < 0
    y = 0;
elseif abs(u) < abs(v)
    y = u;
elseif abs(v) < abs(u)
    y = v;
elseif abs(v) == abs(u)
    y = u;
else
    y = 0;
end

== matlab function O4/Subsystem2/Mass Matrix ==
  data: u input; y output; mI_cart input
function y = fcn(u, mI_cart)

% define mass matrix – assuming negligible mass of structure
m_mp = 0.101; %inertial mass of motor prop
%neglecting mass of structure
mI_cart = (mI_cart/2) - m_mp - 51e-3; %inertial mass without mass of ESC and m_p, structure mass neglected
M = [m_mp, 0;0, mI_cart];


y = M\u;

== matlab function O4/Subsystem2/Relative Displacement ==
  data: u input; y output
function y = fcn(u)

y = u(1) - u(2);

== matlab function O4/Subsystem2/Stiffness Matrix ==
  data: K_11 output; u input; y output size=2
function [K_11,y] = fcn(u)

% define structure characteristics
E = 1.7e9;
I = 2.1992e-10;
L = 0.255;

% define stiffness matrix
K = (E*I)/(L^3) .* [12, -12; -12, 12];

K_11 = K(1,1);

y = K * u;

== matlab function O4/Subsystem1/Reaction Force/MATLAB Function ==
  data: z input; u input; y output
function y = fcn(z,u)

if z <= 0
    if u > 0
        y = u;
    else 
        y = 0;
    end
elseif z >= 1.44
    if u < 0
        y = u;
    else 
        y = 0;
    end
else
    y = 0;
end

== matlab function O4/Subsystem1/Mass & inertia/Mass Parameters ==
  data: mass output
function mass = fcn()

%raw parameters

m_p = 0.15;
m_s = 34.4920e-3;
m_mp = 0.202; %mass of one motor prop
m_ESC = 0.102;
m_cart = 0.4; %mass of one cart without additional stuff


mass = [m_p;m_s;m_mp;m_ESC;m_cart];
